simulink model "egg_incubator"  (R2019a)
settings: Solver=FixedStepAuto  StartTime=0.0  StopTime=300  RelTol=1e-3
undefined symbols (not defined in the file or in its folder): serial
libraries: instrumentlib x3
settings Model: Creator=thotr  LastModifiedBy=thotr

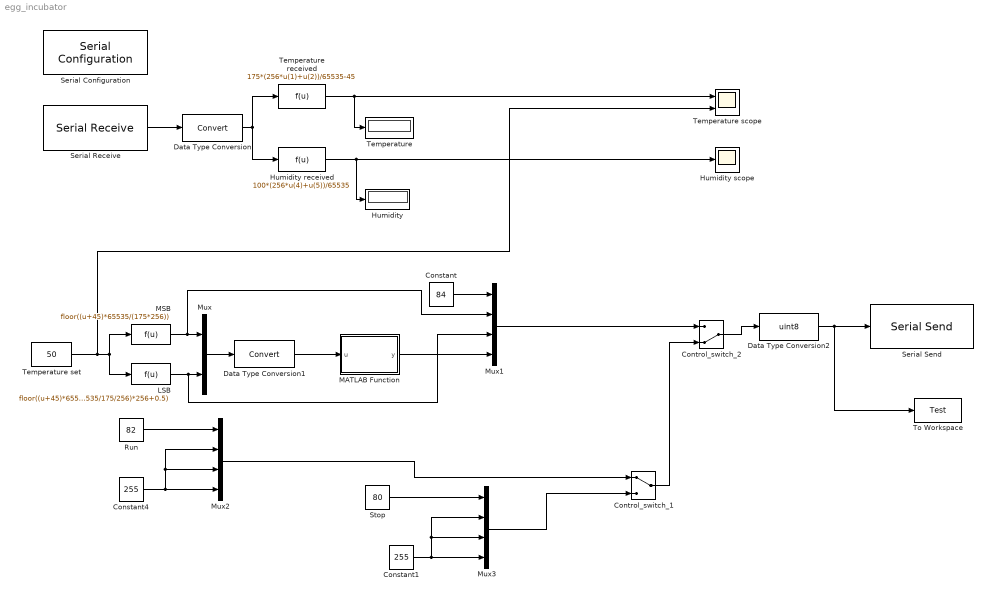
== system egg_incubator ==
  Constant : Constant  Value=84
  Constant1 : Constant  Value=255
  Constant4 : Constant  Value=255
  "Control_switch_1 " : ManualSwitch
  "Control_switch_2 " : ManualSwitch  CurrentSetting=0
  Data Type Conversion : DataTypeConversion  RndMeth=Nearest
  Data Type Conversion1 : DataTypeConversion
  Data Type Conversion2 : DataTypeConversion  OutDataTypeStr=uint8  RndMeth=Nearest
  Humidity : Display
  "Humidity received " : Fcn  Expr=100*(256*u(4)+u(5))/65535
  "Humidity scope " : Scope
  LSB : Fcn  Expr=floor((u+45)*65535/175-floor((u+45)*65535/175/256)*256+0.5)
  MATLAB Function : MATLAB Function  TreatAsAtomicUnit=on
  MSB : Fcn  Expr=floor((u+45)*65535/(175*256))
  Mux : Mux  Inputs=2
  Mux1 : Mux
  Mux2 : Mux
  Mux3 : Mux
  Run : Constant  Value=82
  Serial Configuration : instrumentlib/Serial Configuration  Priority=-200000  ComPortMenu=COM8  ComPort=COM8  ObjConstructor=serial('COM8');  BaudRate=9600  DataBits=8  Parity=none  StopBits=1  FlowControl=none  Timeout=10  ByteOrder=LittleEndian
  Serial Receive : instrumentlib/Serial Receive  ComPortMenu=COM8  ComPort=COM8  ObjConstructor=serial('COM8');  Header=Se  Terminator=<none>  DataSize=9  DataType=uint8  EnableBlockingMode=on  ActionDataUnavailable=Output last received value  CustomValue=0  SampleTime=1
  Serial Send : instrumentlib/Serial Send  ComPortMenu=COM8  ComPort=COM8  ObjConstructor=serial('COM8');  Header=Se  Terminator=En  EnableBlockingMode=on
  Stop : Constant  Value=80
  "Temperature " : Display
  "Temperature received " : Fcn  Expr=175*(256*u(1)+u(2))/65535-45
  "Temperature scope " : Scope  NumInputPorts=2
  "Temperature set " : Constant  Value=50
  To Workspace : ToWorkspace  VariableName=Test  SaveFormat=Timeseries  SampleTime=-1
  wires:
  "Temperature received "/1 -> "Temperature "/1, "Temperature scope "/1
  Serial Receive/1 -> Data Type Conversion/1
  Data Type Conversion/1 -> "Humidity received "/1, "Temperature received "/1
  "Humidity received "/1 -> Humidity/1, "Humidity scope "/1
  "Temperature set "/1 -> "Temperature scope "/2, MSB/1, LSB/1
  MSB/1 -> Mux1/2, Mux/1
  LSB/1 -> Mux1/3, Mux/2
  Mux/1 -> Data Type Conversion1/1
  Constant/1 -> Mux1/1
  MATLAB Function/1(y) -> Mux1/4
  Data Type Conversion2/1 -> To Workspace/1, Serial Send/1
  Mux1/1 -> "Control_switch_2 "/1
  "Control_switch_2 "/1 -> Data Type Conversion2/1
  Run/1 -> Mux2/1
  Constant4/1 -> Mux2/4, Mux2/3, Mux2/2
  Stop/1 -> Mux3/1
  Constant1/1 -> Mux3/4, Mux3/3, Mux3/2
  Mux2/1 -> "Control_switch_1 "/1
  Mux3/1 -> "Control_switch_1 "/2
  "Control_switch_1 "/1 -> "Control_switch_2 "/2
  Data Type Conversion1/1 -> MATLAB Function/1(u)

== matlab function egg_incubator/MATLAB Function ==
  data: u input; y output
function y = crc8(u)
A = uint8([0 1; 0 1]);
B = uint8([0 0; 1 1]);
TTable = bitxor(A, B);
data = uint8([u(1) u(2)]);
polynomial = uint8(49);
polynomial_bin = bitget(polynomial,8:-1:1,'uint8');
crc_initial = uint8(255);
crc_bin = bitget(crc_initial,8:-1:1,'uint8');
 for i=1:2
    data_bin = bitget(data(i),8:-1:1,'uint8');
    crc_bin = bitxor(data_bin, crc_bin, 'uint8');
    for j=1:8
        if (crc_bin(1)==0)
            for k=1:7
                crc_bin(k) = crc_bin(k+1);
            end
            crc_bin(8) = 0;
        else
            for k=1:7
                crc_bin(k) = crc_bin(k+1);
            end
            crc_bin(8) = 0;
            crc_bin = bitxor(crc_bin,polynomial_bin);
        end
    end
 end
crc = uint8(0);
for i=1:8
    crc = crc + crc_bin(i)*2^(8-i);
end
crc_byte = double(crc);
y = crc_byte;
